simulink model "sliding"  (R2016b)
settings: Solver=ode15s  StartTime=0.0  StopTime=10.0  FixedStep=ts  RelTol=1e-4
values from neighbouring files (symbols this model uses):
  b = 0.0167    [script.m]
  J = 0.0167    [script.m]
  Kb = 0.8    [script.m]
  Kt = 0.8    [script.m]
  La = 0.012    [script.m]
  Ra = 0.6    [script.m]
libraries: simulink x1
settings Model: Creator=auralius  LastModifiedBy=Daniel
settings DataIOCC: LimitDataPoints=on  SaveFormat=Array
settings OptimizationCC: BlockReduction=off  BooleanDataType=off  LifeSpan=inf
settings DebuggingCC: SaveWithParameterizedLinksMsg=none  UnderspecifiedInitializationDetection=Classic  MergeDetectMultiDrivingBlocksExec=none  SignalResolutionControl=TryResolveAllWithWarning  SFUnexpectedBacktrackingDiag=warning  SFNoUnconditionalDefaultTransitionDiag=warning  SFExecutionAtInitializationDiag=none
settings HardwareCC: ProdBitPerPointer=32  ProdBitPerSizeT=32  ProdBitPerPtrDiffT=32  ProdLargestAtomicFloat=None  ProdIntDivRoundTo=Undefined  ProdEndianess=Unspecified  ProdWordSize=32  ProdHWDeviceType=32-bit Generic  TargetUnknown=on
settings ModelReferenceCC: PropagateSignalLabelsOutOfModel=off
settings GRTTargetCC: TargetLangStandard=C89/C90 (ANSI)  GeneratePreprocessorConditionals=Disable all
settings ConfigComp: CovMetricSettings=dw  CovHtmlReporting=on  CovSaveCumulativeToWorkspaceVar=on  CovSaveSingleToWorkspaceVar=on  CovExternalEMLEnable=off

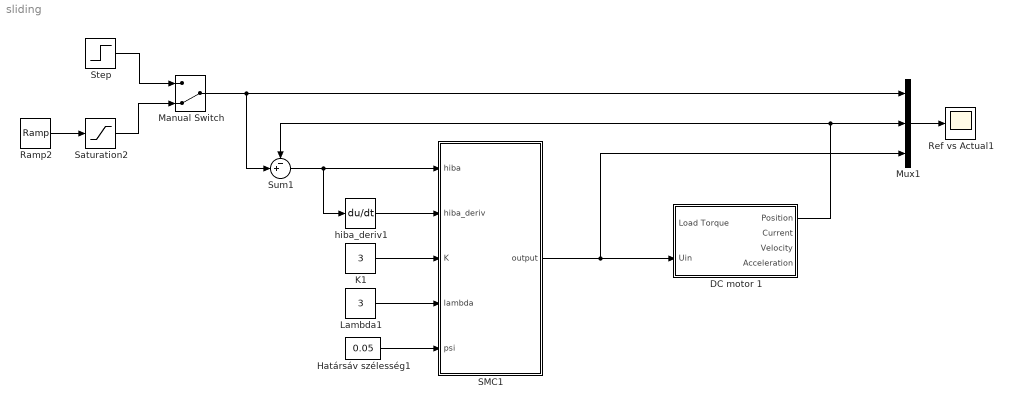
== system sliding ==
  DC motor 1 : Subsystem
  "Határsáv szélesség1 " : Constant  Value=0.05
  K1 : Constant  Value=3
  Lambda1 : Constant  Value=3
  Manual Switch : ManualSwitch  CurrentSetting=0
  Mux1 : Mux  Inputs=3
  Ramp2 : simulink/Sources/Ramp  slope=1000  start=1  X0=0
  Ref vs Actual1 : Scope
  SMC1 : MATLAB Function  TreatAsAtomicUnit=on
  Saturation2 : Saturate  UpperLimit=50  LowerLimit=0
  Step : Step  After=50  SampleTime=0
  Sum1 : Sum  Inputs=-+|
  hiba_deriv1 : Derivative
  wires:
  hiba_deriv1/1 -> SMC1/2(hiba_deriv)
  Sum1/1 -> SMC1/1(hiba), hiba_deriv1/1
  Lambda1/1 -> SMC1/4(lambda)
  K1/1 -> SMC1/3(K)
  "Határsáv szélesség1 "/1 -> SMC1/5(psi)
  Mux1/1 -> Ref vs Actual1/1
  DC motor 1/1("Position ") -> Sum1/1, Mux1/2
  SMC1/1(output) -> Mux1/3, DC motor 1/2("Uin ")
  Ramp2/1 -> Saturation2/1
  Saturation2/1 -> Manual Switch/2
  Step/1 -> Manual Switch/1
  Manual Switch/1 -> Sum1/2, Mux1/1

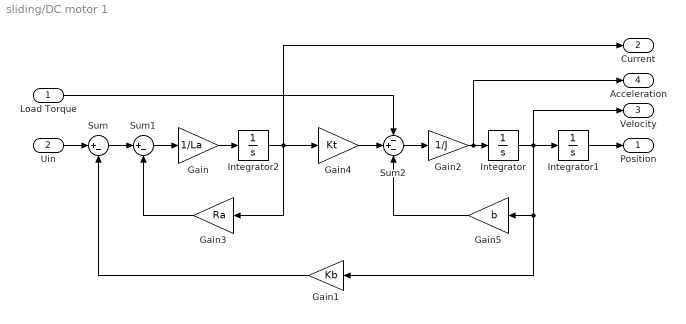
== system sliding/DC motor 1 ==
  Load Torque : Inport
  "Uin " : Inport  Port=2  Interpolate=off
  Gain : Gain  Gain=1/La
  Gain1 : Gain  Gain=Kb
  Gain2 : Gain  Gain=1/J
  Gain3 : Gain  Gain=Ra
  Gain4 : Gain  Gain=Kt
  Gain5 : Gain  Gain=b
  Integrator : Integrator
  Integrator1 : Integrator
  Integrator2 : Integrator  IgnoreLimit=on
  Sum : Sum  Inputs=|+-
  Sum1 : Sum  Inputs=|+-
  Sum2 : Sum  Inputs=-+-
  "Position " : Outport
  Current : Outport  Port=2
  Velocity : Outport  Port=3
  Acceleration : Outport  Port=4
  wires:
  Gain1/1 -> Sum/2
  "Uin "/1 -> Sum/1
  Sum/1 -> Sum1/1
  Sum1/1 -> Gain/1
  Load Torque/1 -> Sum2/1
  Gain3/1 -> Sum1/2
  Gain/1 -> Integrator2/1
  Integrator2/1 -> Current/1, Gain4/1, Gain3/1
  Gain4/1 -> Sum2/2
  Sum2/1 -> Gain2/1
  Gain2/1 -> Acceleration/1, Integrator/1
  Gain5/1 -> Sum2/3
  Integrator/1 -> Integrator1/1, Gain1/1, Gain5/1, Velocity/1
  Integrator1/1 -> "Position "/1

== matlab function sliding/SMC1 ==
  data: hiba input; output output; hiba_deriv input; K input; lambda input; psi input
function output  = smc(hiba, hiba_deriv, K, lambda, psi)
    s = lambda * hiba + hiba_deriv;
    
    if (abs(s) > psi)    
       sat_s = sign(s);
    else
        sat_s = s/psi;
    end
    
    output =  s - K * sat_s;
end
